simulink model "Exp5"  (R2020a)
settings: Solver=VariableStepAuto  StartTime=0.0  StopTime=10  RelTol=1e-3
InitFcn:
  | Voc=32.9;
  | Iscn=8.21;
  | k=1.38e-23;
  | Ns=54;
  | Np=1;
  | G1=800;
  | Gn=1000;
  | Kv=-0.1230;
  | KI=0.0032;
  | T=301;
  | Tn=300;
  | q=1.6e-19;
  | n=1;
  | I0n=9.85e-8;
  | Eg=1.12;
  | Ign=8.214;
  | Rs=0.221;
  | Rp=414.5;
  | a=1.0
libraries: powerlib x17, powerlib_meascontrol x5, simulink x2
settings Model: Creator=ahmed  LastModifiedBy=ahmed

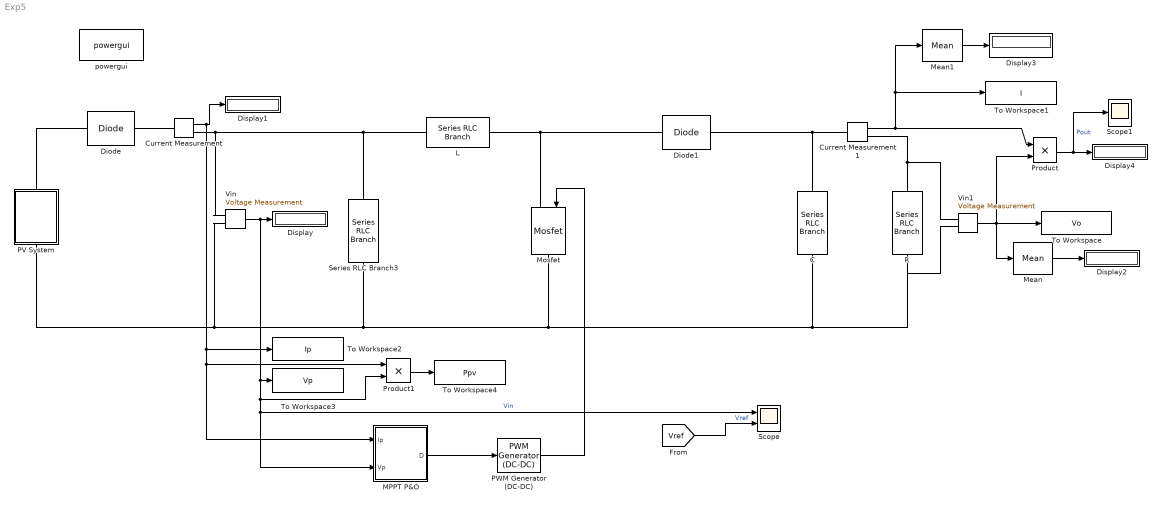
== system Exp5 ==
  C : powerlib/Elements/Series RLC Branch  LConnTagsString=__new0  RConnTagsString=__new0  BranchType=C  Resistance=1  Inductance=1e-3  SetiL0=off  InitialCurrent=0  Capacitance=110e-6  Setx0=off  InitialVoltage=0  Measurements=None
  Current Measurement : powerlib/Measurements/Current Measurement  PhasorSimulation=off  OutputType=Complex  PSBequivalent=0
  Current Measurement1 : powerlib/Measurements/Current Measurement  PhasorSimulation=off  OutputType=Complex  PSBequivalent=0
  Diode : powerlib/Power Electronics/Diode  Ron=0.001  Lon=0  Vf=0.8  IC=0  UseSnubber=0  Rs=500  Cs=250e-9  Measurements=off
  Diode1 : powerlib/Power Electronics/Diode  Ron=0.001  Lon=0  Vf=0.8  IC=0  UseSnubber=0  Rs=500  Cs=250e-9  Measurements=off
  Display{,1..4} (5 alike) : Display
  L : powerlib/Elements/Series RLC Branch  LConnTagsString=__new0  RConnTagsString=__new0  BranchType=L  Resistance=1  Inductance=0.01025  SetiL0=off  InitialCurrent=0  Capacitance=1e-6  Setx0=off  InitialVoltage=0  Measurements=None
  MPPT P&O : Subsystem
  Mean : powerlib_meascontrol/Measurements/Mean  Freq=60  Vinit=0  Ts=0
  Mean1 : powerlib_meascontrol/Measurements/Mean  Freq=60  Vinit=0  Ts=0
  Mosfet : powerlib/Power Electronics/Mosfet  Ron=0.1  Lon=0  Rd=0.01  Vfd=0  IC=0  Rs=1e5  Cs=inf  Measurements=off
  PV System : Subsystem
  PWM Generator (DC-DC) : powerlib_meascontrol/Pulse & Signal Generators/PWM Generator (DC-DC)  Fsw=5000  Ts=0
  Product : Product
  Product1 : Product
  R : powerlib/Elements/Series RLC Branch  LConnTagsString=__new0  RConnTagsString=__new0  BranchType=R  Resistance=25.5  Inductance=1e-3  SetiL0=off  InitialCurrent=0  Capacitance=1e-6  Setx0=off  InitialVoltage=0  Measurements=None
  Scope : Scope  NumInputPorts=2
  Scope1 : Scope
  Series RLC Branch3 : powerlib/Elements/Series RLC Branch  LConnTagsString=__new0  RConnTagsString=__new0  BranchType=C  Resistance=1  Inductance=1e-3  SetiL0=off  InitialCurrent=0  Capacitance=110e-6  Setx0=off  InitialVoltage=0  Measurements=None
  To Workspace : ToWorkspace  VariableName=Vo  SampleTime=-1
  To Workspace1 : ToWorkspace  VariableName=I  SampleTime=-1
  To Workspace2 : ToWorkspace  VariableName=Ip  SampleTime=-1
  To Workspace3 : ToWorkspace  VariableName=Vp  SampleTime=-1
  To Workspace4 : ToWorkspace  VariableName=Ppv  SampleTime=-1
  Vin : powerlib/Measurements/Voltage Measurement  PhasorSimulation=off  OutputType=Complex  PSBequivalent=0
  Vin1 : powerlib/Measurements/Voltage Measurement  PhasorSimulation=off  OutputType=Complex  PSBequivalent=0
  powergui : powerlib/powergui  Priority=1  SimulationMode=Continuous  SampleTime=50e-6  frequency=60  Iterations=50  frequencyindice=0  Pbase=100e6  ErrMax=1e-4  UnitsV=kV  UnitsW=MW  buscounter=0  FunctionMessages=off  echomessages=off  EnableUseOfTLC=off  CurrentSourceSwitches=off  DisableSnubberDevices=off  DisableRonSwitches=off  DisableVfSwitches=off  DisplayEquations=off  AutomaticDiscreteSolvers=off  SolverType=Tustin/Backward Euler (TBE)  Interpol=off  ExternalGateDelay=off  methode=off  Ts=100  x0status=blocks  SPID=on  SwTol=0  HookPort=off  NonlinearTolerance=1e-4  nMaxIteration=100  ContinueOnMaxIteration=off  RestoreLinks=warning  ResistiveCurrentMeasurement=off  Frange=[0:2:500]  Ylog=off  Xlog=on  ShowGrid=off  save=off  variable=ZData  structure=0  ZoomFFT=off  StartTime=0.0  cycles=1  DisplayStyle=1  fundamental=60  FreqAxis=off  MaxFrequency=1000  frequencyindicesteady=1  RmsSteady=1  display=off
  wires:
  Vin/1 -> To Workspace3/1, Product1/2, MPPT P&O/2(Vp), Scope/1, Display/1  "Vin"
  Current Measurement/1 -> To Workspace2/1, Product1/1, MPPT P&O/1(Ip), Display1/1
  Vin1/1 -> Product/2, To Workspace/1, Mean/1
  Mean/1 -> Display2/1
  Current Measurement1/1 -> To Workspace1/1, Mean1/1, Product/1
  Mean1/1 -> Display3/1
  MPPT P&O/1(D) -> PWM Generator (DC-DC)/1
  PWM Generator (DC-DC)/1 -> Mosfet/1
  [Vref] -> Scope/2  "Vref"
  Product/1 -> Scope1/1, Display4/1  "Pout"
  Product1/1 -> To Workspace4/1
  connections:
  Diode/RConn1 -- Current Measurement/LConn1
  Diode/LConn1 -- PV System/RConn1
  L/LConn1 -- Vin/LConn1 -- Current Measurement/RConn1 -- Series RLC Branch3/LConn1
  Mosfet/LConn1 -- Diode1/LConn1 -- L/RConn1
  PV System/LConn1 -- Vin/LConn2 -- Series RLC Branch3/RConn1 -- Mosfet/RConn1 -- Vin1/LConn2 -- R/RConn1 -- C/RConn1
  Diode1/RConn1 -- Current Measurement1/LConn1 -- C/LConn1
  Current Measurement1/RConn1 -- Vin1/LConn1 -- R/LConn1

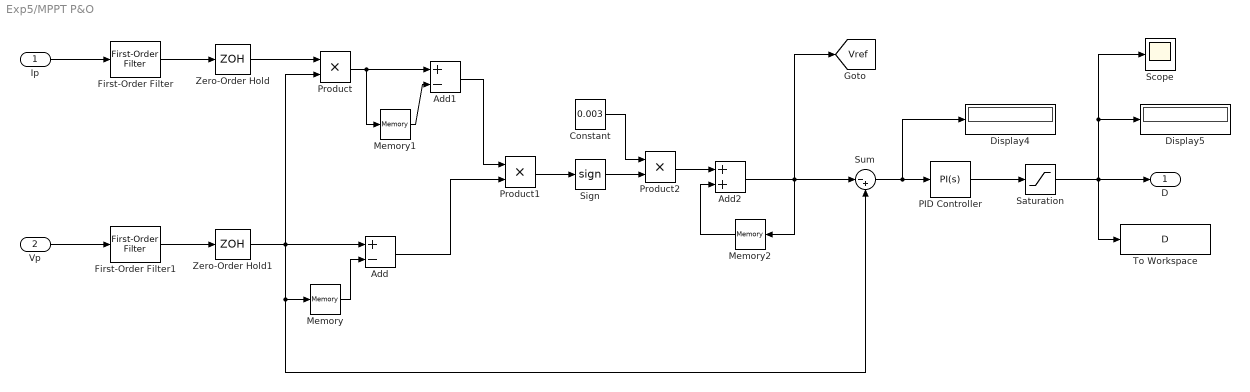
== system Exp5/MPPT P&O ==
  Ip : Inport
  Vp : Inport  Port=2
  Add : Sum  Inputs=+-
  Add1 : Sum  Inputs=+-
  Add2 : Sum
  Constant : Constant  Value=0.003
  Display4 : Display
  Display5 : Display
  First-Order Filter : powerlib_meascontrol/Filters/First-Order Filter  FilterType=Lowpass  Tc=10e-3  Ts=5e-5  Initialize=on  Vac_Init=[0, 0, 60]  Vdc_Init=0  PlotResponse=off  FreqRange="[0,  200,  1]"
  First-Order Filter1 : powerlib_meascontrol/Filters/First-Order Filter  FilterType=Lowpass  Tc=10e-3  Ts=5e-5  Initialize=on  Vac_Init=[0, 0, 60]  Vdc_Init=0  PlotResponse=off  FreqRange="[0,  200,  1]"
  Memory : Memory
  Memory1 : Memory
  Memory2 : Memory
  PID Controller : simulink/Continuous/PID Controller  Controller=PI  Form=Parallel  TimeDomain=Continuous-time  UseExternalTs=off  SampleTime=-1  IntegratorMethod=Forward Euler  FilterMethod=Forward Euler  ControllerParametersSource=internal  P=0.001  I=0.1  D=0  UseFilter=on  N=100  TunerSelectOption=Transfer Function Based (PID Tuner App)  InitialConditionSource=internal  InitialConditionForIntegrator=0  InitialConditionForFilter=0  DifferentiatorICPrevScaledInput=0  ExternalReset=none  TrackingMode=off  Kt=1  LimitOutput=off  UpperSaturationLimit=inf  LowerSaturationLimit=-inf  LinearizeAsGain=on  AntiWindupMode=none  Kb=1  POutMin=[]  POutMax=[]  IOutMin=[]  IOutMax=[]  DOutMin=[]  DOutMax=[]  NOutMin=[]  NOutMax=[]  SumOutMin=[]  SumOutMax=[]  SaturationOutMin=[]  SaturationOutMax=[]  PParamMin=[]  PParamMax=[]  IParamMin=[]  IParamMax=[]  DParamMin=[]  DParamMax=[]  NParamMin=[]  NParamMax=[]  KbParamMin=[]  KbParamMax=[]  KtParamMin=[]  KtParamMax=[]  KbOutMin=[]  KbOutMax=[]  KtOutMin=[]  KtOutMax=[]  IntegratorOutMin=[]  IntegratorOutMax=[]  FilterOutMin=[]  FilterOutMax=[]  SumI1OutMin=[]  SumI1OutMax=[]  SumI2OutMin=[]  SumI2OutMax=[]  SumI3OutMin=[]  SumI3OutMax=[]  SumI4OutMin=[]  SumI4OutMax=[]  SumDOutMin=[]  SumDOutMax=[]  DifferentiatorOutMin=[]  DifferentiatorOutMax=[]  FilterDiffOutCoefMin=[]  FilterDiffOutCoefMax=[]  ReciprocalOutMin=[]  ReciprocalOutMax=[]  SumDenOutMin=[]  SumDenOutMax=[]  SumNumOutMin=[]  SumNumOutMax=[]  DivideOutMin=[]  DivideOutMax=[]  UdiffTsProdOutMin=[]  UdiffTsProdOutMax=[]  NTsProdOutMin=[]  NTsProdOutMax=[]  UintegralTsProdOutMin=[]  UintegralTsProdOutMax=[]  UngainTsProdOutMin=[]  UngainTsProdOutMax=[]  IntegratorContinuousStateAttributes=''  IntegratorStateMustResolveToSignalObject=off  IntegratorRTWStateStorageClass=Auto  FilterContinuousStateAttributes=''  FilterStateMustResolveToSignalObject=off  FilterRTWStateStorageClass=Auto  ParallelPVariant=InternalParameters  IdealPVariant=Disabled  IVariant=InternalParameters  DVariant=Disabled  IntegratorVariant=Continuous  SatVariant=Disabled  AWVariant=Passthrough  PCopyVariant=Disabled  TRVariant=Disabled  FdbkBlocksVariant=Forward  IdealPFdbkVariant=Disabled  SatFdbkVariant=Disabled  DerivativeFilterVariant=Disabled  NVariant=Disabled  NCopyVariant=Disabled_SignalSpec  FilterICVariant=Disabled  IntegratorICVariant=InternalICs  ExternalResetVariant=Disabled  TRSumVariant=Passthrough  SumFdbkVariant=Disabled  SumVariant=Sum_PI  TsampFilterVariant=InternalTs  TsampNgainVariant=Passthrough  TsampIntegralVariant=Passthrough
  Product : Product
  Product1 : Product
  Product2 : Product
  Saturation : Saturate  UpperLimit=1  LowerLimit=0
  Scope : Scope
  Sign : Signum
  Sum : Sum  Inputs=|-+
  To Workspace : ToWorkspace  VariableName=D  SaveFormat=Timeseries  SampleTime=-1
  Zero-Order Hold : ZeroOrderHold  SampleTime=0.0001
  Zero-Order Hold1 : ZeroOrderHold  SampleTime=0.0001
  D : Outport
  tag scope: Vref=global
  wires:
  Add2/1 -> Memory2/1, [Vref], Sum/1
  Zero-Order Hold1/1 -> Memory/1, Sum/2, Product/2, Add/1
  Saturation/1 -> To Workspace/1, D/1, Display5/1, Scope/1
  Product2/1 -> Add2/1
  Sum/1 -> Display4/1, PID Controller/1
  Sign/1 -> Product2/2
  Add1/1 -> Product1/1
  Memory1/1 -> Add1/2
  First-Order Filter1/1 -> Zero-Order Hold1/1
  PID Controller/1 -> Saturation/1
  Memory2/1 -> Add2/2
  Add/1 -> Product1/2
  Product/1 -> Memory1/1, Add1/1
  Constant/1 -> Product2/1
  Memory/1 -> Add/2
  Vp/1 -> First-Order Filter1/1
  First-Order Filter/1 -> Zero-Order Hold/1
  Product1/1 -> Sign/1
  Zero-Order Hold/1 -> Product/1
  Ip/1 -> First-Order Filter/1

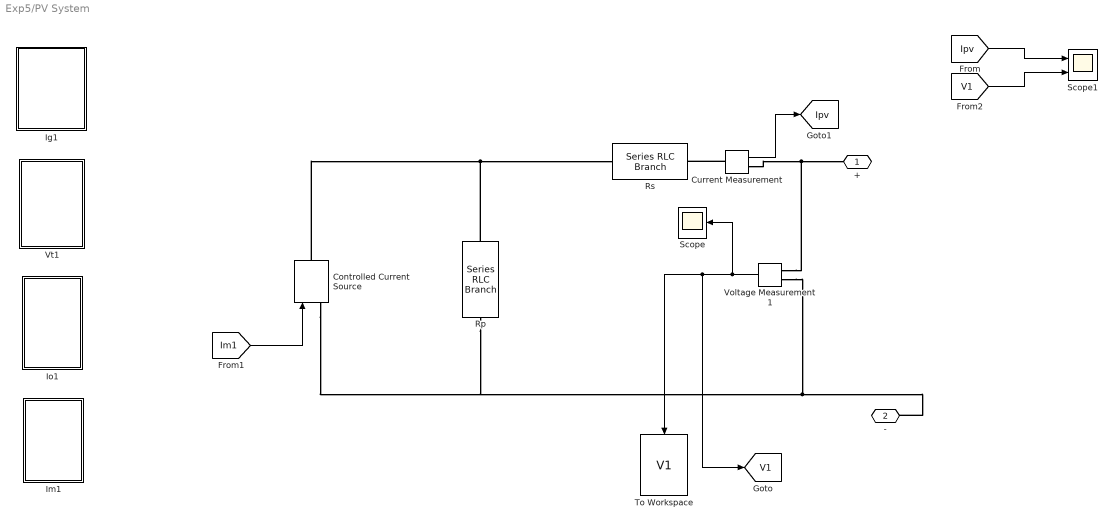
== system Exp5/PV System ==
  Controlled Current Source : powerlib/Electrical Sources/Controlled Current Source  Initialize=on  Source_Type=AC  Amplitude=0  Phase=0  Frequency=0  Measurements=None
  Current Measurement : powerlib/Measurements/Current Measurement  PhasorSimulation=off  OutputType=Complex  PSBequivalent=0
  Ig1 : Subsystem
  Im1 : Subsystem
  Io1 : Subsystem
  Rp : powerlib/Elements/Series RLC Branch  LConnTagsString=__new0  RConnTagsString=__new0  BranchType=R  Resistance=Rp  Inductance=1e-3  SetiL0=off  InitialCurrent=0  Capacitance=1e-6  Setx0=off  InitialVoltage=0  Measurements=None
  Rs : powerlib/Elements/Series RLC Branch  LConnTagsString=__new0  RConnTagsString=__new0  BranchType=R  Resistance=Rs  Inductance=1e-3  SetiL0=off  InitialCurrent=0  Capacitance=1e-6  Setx0=off  InitialVoltage=0  Measurements=None
  Scope : Scope
  Scope1 : Scope  NumInputPorts=2
  To Workspace : ToWorkspace  VariableName=V1  SaveFormat=Timeseries  SampleTime=-1
  Voltage Measurement1 : powerlib/Measurements/Voltage Measurement  PhasorSimulation=off  OutputType=Complex  PSBequivalent=0
  Vt1 : Subsystem
  + : PMIOPort  Side=Right
  - : PMIOPort  Port=2  Side=Left
  tag scope: Ipv=global, V1=global
  wires:
  [Im1] -> Controlled Current Source/1
  Voltage Measurement1/1 -> [V1], To Workspace/1, Scope/1
  Current Measurement/1 -> [Ipv]
  [Ipv] -> Scope1/1
  [V1] -> Scope1/2
  connections:
  Voltage Measurement1/LConn1 -- Current Measurement/RConn1 -- +/RConn1
  Voltage Measurement1/LConn2 -- Controlled Current Source/LConn1 -- Rp/RConn1 -- -/RConn1
  Rp/LConn1 -- Controlled Current Source/RConn1 -- Rs/LConn1
  Current Measurement/LConn1 -- Rs/RConn1

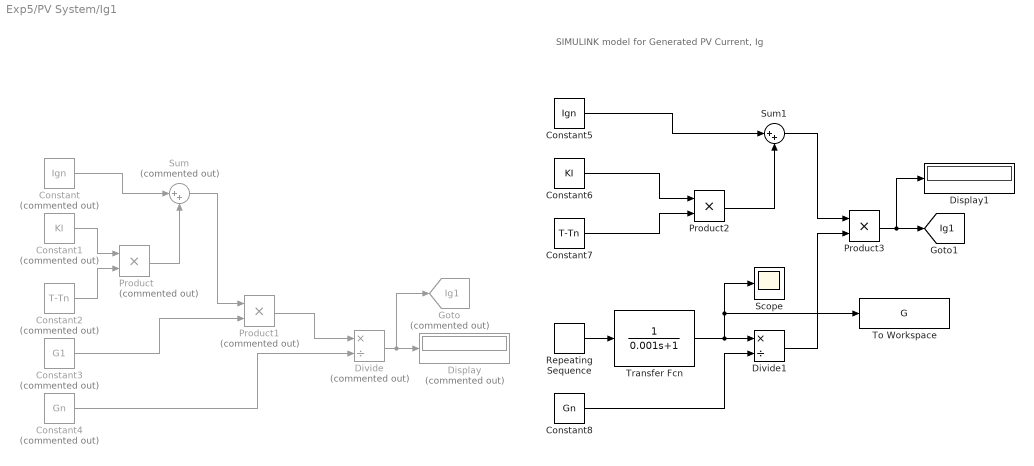
== system Exp5/PV System/Ig1 ==
  note: SIMULINK model for Generated PV Current, Ig
  Constant : Constant  Commented=on  Value=Ign
  Constant1 : Constant  Commented=on  Value=KI
  Constant2 : Constant  Commented=on  Value=T-Tn
  Constant3 : Constant  Commented=on  Value=G1
  Constant4 : Constant  Commented=on  Value=Gn
  Constant5 : Constant  Value=Ign
  Constant6 : Constant  Value=KI
  Constant7 : Constant  Value=T-Tn
  Constant8 : Constant  Value=Gn
  Display : Display  Commented=on
  Display1 : Display
  Divide : Product  Commented=on  Inputs=*/
  Divide1 : Product  Inputs=*/
  Goto : Goto  Commented=on  GotoTag=Ig1  TagVisibility=global
  Product : Product  Commented=on
  Product1 : Product  Commented=on
  Product2 : Product
  Product3 : Product
  Repeating Sequence : simulink/Sources/Repeating Sequence  rep_seq_t=[0 3 3.1 7 7.1 10]  rep_seq_y=[640 640 810 810 980 980]
  Scope : Scope
  Sum : Sum  Commented=on  Inputs=|++
  Sum1 : Sum  Inputs=|++
  To Workspace : ToWorkspace  VariableName=G  SaveFormat=Timeseries  SampleTime=-1
  Transfer Fcn : TransferFcn  Denominator=[0.001 1]
  tag scope: Ig1=global
  wires:
  Divide/1 -> Goto/1, Display/1
  Product1/1 -> Divide/1
  Constant1/1 -> Product/1
  Constant/1 -> Sum/1
  Product/1 -> Sum/2
  Constant2/1 -> Product/2
  Constant3/1 -> Product1/2
  Sum/1 -> Product1/1
  Constant4/1 -> Divide/2
  Repeating Sequence/1 -> Transfer Fcn/1
  Constant5/1 -> Sum1/1
  Constant6/1 -> Product2/1
  Constant7/1 -> Product2/2
  Transfer Fcn/1 -> To Workspace/1, Scope/1, Divide1/1
  Constant8/1 -> Divide1/2
  Product2/1 -> Sum1/2
  Divide1/1 -> Product3/2
  Sum1/1 -> Product3/1
  Product3/1 -> Display1/1, [Ig1]

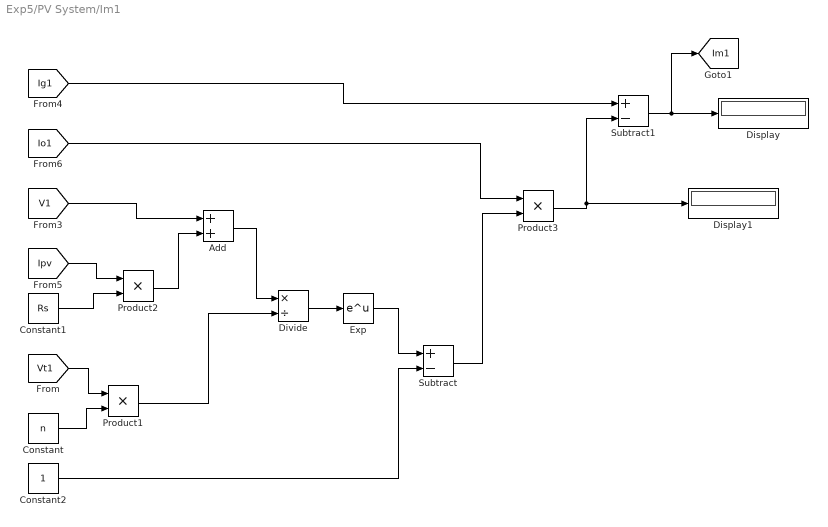
== system Exp5/PV System/Im1 ==
  Add : Sum
  Constant : Constant  Value=n
  Constant1 : Constant  Value=Rs
  Constant2 : Constant
  Display : Display
  Display1 : Display
  Divide : Product  Inputs=*/
  Exp : Math  SaturateOnIntegerOverflow=on
  Product1 : Product
  Product2 : Product
  Product3 : Product
  Subtract : Sum  Inputs=+-
  Subtract1 : Sum  Inputs=+-
  tag scope: Im1=global
  wires:
  Exp/1 -> Subtract/1
  Product2/1 -> Add/2
  [Vt1] -> Product1/1
  [Ig1] -> Subtract1/1
  Constant1/1 -> Product2/2
  Subtract1/1 -> [Im1], Display/1
  Add/1 -> Divide/1
  [Ipv] -> Product2/1
  Product1/1 -> Divide/2
  [V1] -> Add/1
  [Io1] -> Product3/1
  Divide/1 -> Exp/1
  Constant2/1 -> Subtract/2
  Subtract/1 -> Product3/2
  Product3/1 -> Display1/1, Subtract1/2
  Constant/1 -> Product1/2

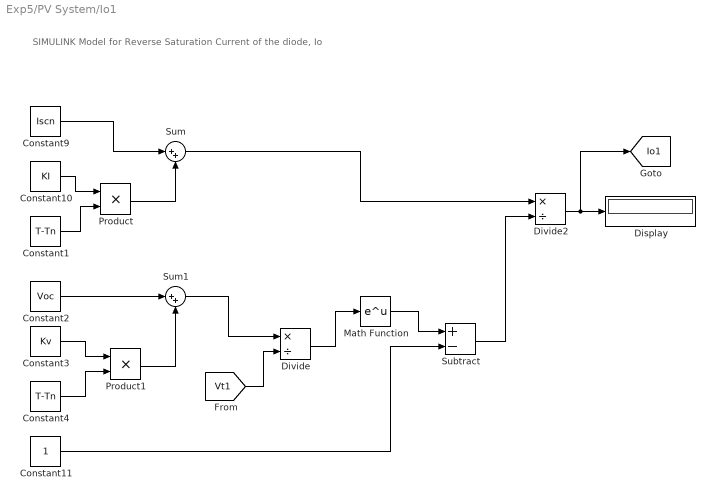
== system Exp5/PV System/Io1 ==
  note: SIMULINK Model for Reverse Saturation Current of the diode, Io
  Constant1 : Constant  Value=T-Tn
  Constant10 : Constant  Value=KI
  Constant11 : Constant
  Constant2 : Constant  Value=Voc
  Constant3 : Constant  Value=Kv
  Constant4 : Constant  Value=T-Tn
  Constant9 : Constant  Value=Iscn
  Display : Display
  Divide : Product  Inputs=*/
  Divide2 : Product  Inputs=*/
  Math Function : Math  SaturateOnIntegerOverflow=on
  Product : Product
  Product1 : Product
  Subtract : Sum  Inputs=+-
  Sum : Sum  Inputs=|++
  Sum1 : Sum  Inputs=|++
  tag scope: Io1=global
  wires:
  Constant4/1 -> Product1/2
  [Vt1] -> Divide/2
  Product/1 -> Sum/2
  Math Function/1 -> Subtract/1
  Sum/1 -> Divide2/1
  Constant9/1 -> Sum/1
  Product1/1 -> Sum1/2
  Constant11/1 -> Subtract/2
  Constant3/1 -> Product1/1
  Sum1/1 -> Divide/1
  Divide2/1 -> [Io1], Display/1
  Constant10/1 -> Product/1
  Subtract/1 -> Divide2/2
  Constant2/1 -> Sum1/1
  Divide/1 -> Math Function/1
  Constant1/1 -> Product/2

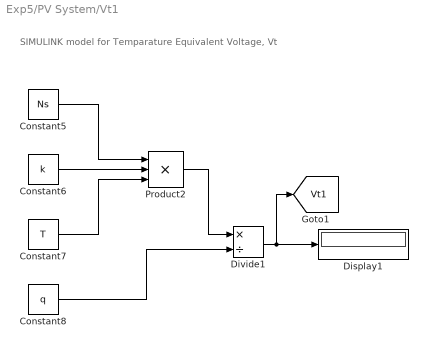
== system Exp5/PV System/Vt1 ==
  note: SIMULINK model for Temparature Equivalent Voltage, Vt
  Constant5 : Constant  Value=Ns
  Constant6 : Constant  Value=k
  Constant7 : Constant  Value=T
  Constant8 : Constant  Value=q
  Display1 : Display
  Divide1 : Product  Inputs=*/
  Product2 : Product  Inputs=3
  tag scope: Vt1=global
  wires:
  Product2/1 -> Divide1/1
  Divide1/1 -> [Vt1], Display1/1
  Constant5/1 -> Product2/1
  Constant7/1 -> Product2/3
  Constant8/1 -> Divide1/2
  Constant6/1 -> Product2/2
